simulink model "Tavola3_3ordine"  (R2018b)
settings: Solver=FixedStepAuto  StartTime=0.0  StopTime=70  RelTol=1e-3
libraries: simulink x1
settings Model: Creator=Utente  LastModifiedBy=giga4

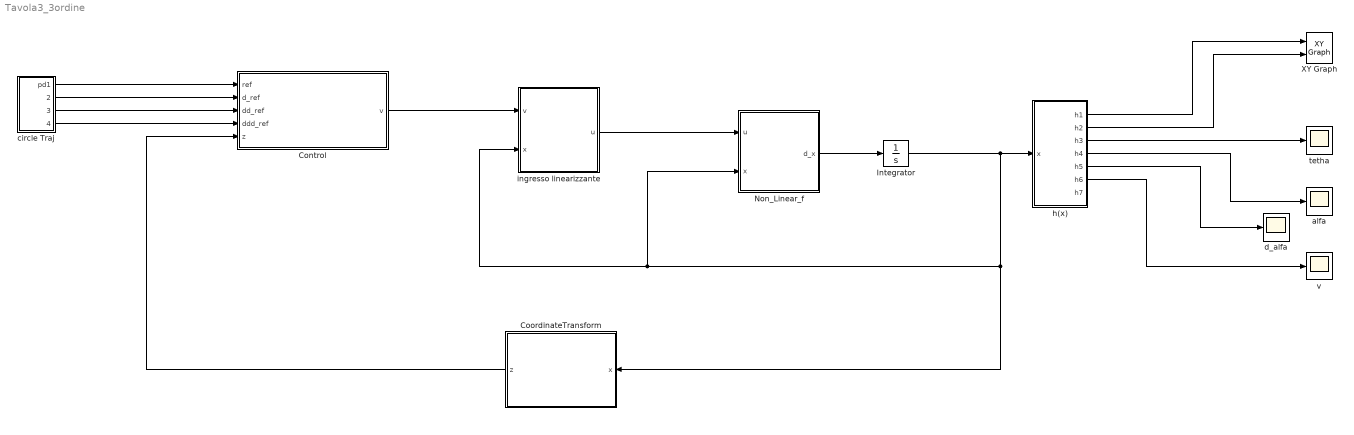
== system Tavola3_3ordine ==
  Control : MATLAB Function  TreatAsAtomicUnit=on
  CoordinateTransform : MATLAB Function  TreatAsAtomicUnit=on
  Integrator : Integrator  InitialCondition=[0,0,pi/2,0.017,0,5,0]
  "Non_Linear_f " : MATLAB Function  TreatAsAtomicUnit=on
  XY Graph : simulink/Sinks/XY Graph  xmin=-100  xmax=100  ymin=-100  ymax=100  st=-1
  alfa : Scope
  circle Traj : Subsystem
  d_alfa : Scope
  h(x) : MATLAB Function  TreatAsAtomicUnit=on
  ingresso linearizzante : MATLAB Function  TreatAsAtomicUnit=on
  tetha : Scope
  v : Scope
  wires:
  "Non_Linear_f "/1(d_x) -> Integrator/1
  Integrator/1 -> "Non_Linear_f "/2(x), ingresso linearizzante/2(x), CoordinateTransform/1(x), h(x)/1(x)
  ingresso linearizzante/1(u) -> "Non_Linear_f "/1(u)
  h(x)/3(h3) -> tetha/1
  h(x)/4(h4) -> alfa/1
  h(x)/1(h1) -> XY Graph/1
  h(x)/2(h2) -> XY Graph/2
  h(x)/6(h6) -> v/1
  Control/1(v) -> ingresso linearizzante/1(v)
  CoordinateTransform/1(z) -> Control/5(z)
  h(x)/5(h5) -> d_alfa/1
  circle Traj/1(pd1) -> Control/1(ref)
  circle Traj/2(d_pd1) -> Control/2(d_ref)
  circle Traj/3(dd_pd) -> Control/3(dd_ref)
  circle Traj/4(ddd_pd) -> Control/4(ddd_ref)

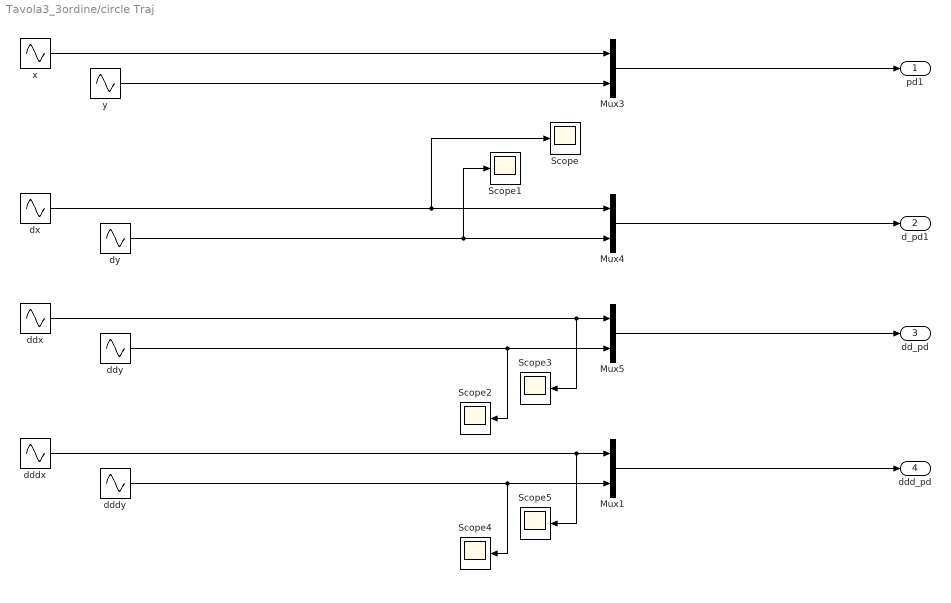
== system Tavola3_3ordine/circle Traj ==
  Mux{1,3..5} (4 alike) : Mux  Inputs=2
  Scope{,1..5} (6 alike) : Scope
  dddx : Sin  Amplitude=10  SampleTime=0
  dddy : Sin  Amplitude=-10  Phase=pi/2  SampleTime=0
  ddx : Sin  Amplitude=-10  Phase=pi/2  SampleTime=0
  ddy : Sin  Amplitude=-10  SampleTime=0
  dx : Sin  Amplitude=-10  SampleTime=0
  dy : Sin  Amplitude=10  Phase=pi/2  SampleTime=0
  x : Sin  Amplitude=10  Phase=pi/2  SampleTime=0
  y : Sin  Amplitude=10  SampleTime=0
  pd1 : Outport
  d_pd1 : Outport  Port=2
  dd_pd : Outport  Port=3
  ddd_pd : Outport  Port=4
  wires:
  ddx/1 -> Scope3/1, Mux5/1
  Mux3/1 -> pd1/1
  x/1 -> Mux3/1
  dddy/1 -> Scope4/1, Mux1/2
  ddy/1 -> Scope2/1, Mux5/2
  Mux1/1 -> ddd_pd/1
  dx/1 -> Scope/1, Mux4/1
  dy/1 -> Scope1/1, Mux4/2
  Mux5/1 -> dd_pd/1
  y/1 -> Mux3/2
  dddx/1 -> Scope5/1, Mux1/1
  Mux4/1 -> d_pd1/1

== matlab function Tavola3_3ordine/h(x) ==
  data: x input; h1 output; h2 output; h3 output; h4 output; h5 output; h6 output; h7 output
function [h1,h2,h3,h4,h5,h6,h7] = h(x)

x1 = x(1);
x2 = x(2);
x3 = x(3);
x4 = x(4);
x5 = x(5);
x6 = x(6);
x7 = x(7);


h1 = x1;
h2 = x2;
h3 = x3;
h4 = x4;
h5 = x5;
h6 = x6;
h7 = x7;

== matlab function Tavola3_3ordine/Non_Linear_f  ==
  data: u input; d_x output; x input
function d_x = statespacef(u,x)

x1 = x(1);
x2 = x(2);
x3 = x(3);
x4 = x(4);
x5 = x(5);
x6 = x(6);
x7 = x(7);


f =                                                                                                                               [x6*cos(x3);
                                                                                                                                  x6*sin(x3);
                                                                                                                                          x7;
                                                                                                                                          x5;
 (2.39*sin(2.0*x4)*x5^2)/(4.79*cos(x4)^2 - 12.5) - (173.0*sin(x4))/(4.79*cos(x4)^2 - 12.5) - (3.28*x7^2*sin(2.0*x4))/(4.79*cos(x4)^2 - 12.5);
       (1.99*sin(3.0*x4) - 6.77*sin(x4))*x7^2 + (23.5*sin(2.0*x4))/(4.79*cos(x4)^2 - 12.5) - (2.19*x5^2*sin(2.0*x4))/(4.79*cos(x4)^2 - 12.5);
                                       (0.547*x6*x7*sin(x4))/(0.228*cos(x4)^2 - 0.315) + (0.228*x5*x7*sin(2.0*x4))/(0.228*cos(x4)^2 - 0.315)];
g1 = [                                              0;
                                                    0;
                                                    0;
                                                    0;
        (2.19*cos(x3) + 3.11)/(4.79*cos(x4)^2 - 12.5);
 -(1.0*(0.547*cos(x4) + 1.0))/(4.79*cos(x4)^2 - 12.5);
                      -0.05/(0.228*cos(x4)^2 - 0.315);];
 
g2 = [                                              0;
                                                    0;
                                                    0;
                                                    0;
        (2.19*cos(x3) + 3.11)/(4.79*cos(x4)^2 - 12.5);
 -(1.0*(0.547*cos(x4) + 1.0))/(4.79*cos(x4)^2 - 12.5);
                       0.05/(0.228*cos(x4)^2 - 0.315)];
d_x = f + [g1,g2]*u;

== matlab function Tavola3_3ordine/ingresso linearizzante ==
  data: v input; u output; x input
function u = inputLinearizzante(v,x)

x1 = x(1);
x2 = x(2);
x3 = x(3);
x4 = x(4);
x5 = x(5);
x6 = x(6);
x7 = x(7);

inv_E =  [                                                                                                                                                                                     -(1.0*cos(x3)*(0.547*cos(x4) + 1.0))/(4.79*cos(x4)^2 - 12.5),                                                                                                                                                                                     -(1.0*cos(x3)*(0.547*cos(x4) + 1.0))/(4.79*cos(x4)^2 - 12.5);
          - (0.05*(x6*cos(x3) + 2*x7*sin(x3)*(1.99*sin(3.0*x4) - 6.77*sin(x4))))/(0.228*cos(x4)^2 - 0.315) - (1.0*x7*cos(x3)*(0.547*cos(x4) + 1.0))/(4.79*cos(x4)^2 - 12.5) - (4.38*x5*sin(2.0*x4)*sin(x3)*(2.19*cos(x3) + 3.11))/(4.79*cos(x4)^2 - 12.5)^2, (0.05*(x6*cos(x3) + 2*x7*sin(x3)*(1.99*sin(3.0*x4) - 6.77*sin(x4))))/(0.228*cos(x4)^2 - 0.315) - (1.0*x7*cos(x3)*(0.547*cos(x4) + 1.0))/(4.79*cos(x4)^2 - 12.5) - (4.38*x5*sin(2.0*x4)*sin(x3)*(2.19*cos(x3) + 3.11))/(4.79*cos(x4)^2 - 12.5)^2];
       
Gamma =  [                                                                                                                                                                                                                                                                                                                                                                                                                                                                                                                                                                                                                                                                                                                                                                                                                         cos(x3)*((1.99*sin(3.0*x4) - 6.77*sin(x4))*x7^2 + (23.5*sin(2.0*x4))/(4.79*cos(x4)^2 - 12.5) - (2.19*x5^2*sin(2.0*x4))/(4.79*cos(x4)^2 - 12.5)) - x6*x7*sin(x3);
 ((0.547*x6*x7*sin(x4))/(0.228*cos(x4)^2 - 0.315) + (0.228*x5*x7*sin(2.0*x4))/(0.228*cos(x4)^2 - 0.315))*(x6*cos(x3) + 2*x7*sin(x3)*(1.99*sin(3.0*x4) - 6.77*sin(x4))) + x7*(cos(x3)*((1.99*sin(3.0*x4) - 6.77*sin(x4))*x7^2 + (23.5*sin(2.0*x4))/(4.79*cos(x4)^2 - 12.5) - (2.19*x5^2*sin(2.0*x4))/(4.79*cos(x4)^2 - 12.5)) - x6*x7*sin(x3)) + x5*sin(x3)*(x7^2*(5.98*cos(3.0*x4) - 6.77*cos(x4)) + (46.9*cos(2.0*x4))/(4.79*cos(x4)^2 - 12.5) - (4.38*x5^2*cos(2.0*x4))/(4.79*cos(x4)^2 - 12.5) + (225.0*sin(2.0*x4)*cos(x4)*sin(x4))/(4.79*cos(x4)^2 - 12.5)^2 - (21.0*x5^2*sin(2.0*x4)*cos(x4)*sin(x4))/(4.79*cos(x4)^2 - 12.5)^2) + x7*cos(x3)*((1.99*sin(3.0*x4) - 6.77*sin(x4))*x7^2 + (23.5*sin(2.0*x4))/(4.79*cos(x4)^2 - 12.5) - (2.19*x5^2*sin(2.0*x4))/(4.79*cos(x4)^2 - 12.5)) + (4.38*x5*sin(2.0*x4)*sin(x3)*((3.28*sin(2.0*x4)*x7^2)/(4.79*cos(x4)^2 - 12.5) + (173.0*sin(x4))/(4.79*cos(x4)^2 - 12.5) - (2.39*x5^2*sin(2.0*x4))/(4.79*cos(x4)^2 - 12.5)))/(4.79*cos(x4)^2 - 12.5)];

 
 u = -inv_E*Gamma+inv_E*v;

== matlab function Tavola3_3ordine/CoordinateTransform ==
  data: z output; x input
function z = transformCoordinate(x)

x1 = x(1);
x2 = x(2);
x3 = x(3);
x4 = x(4);
x5 = x(5);
x6 = x(6);
x7 = x(7);

z =   [                                                                                                                                                       x1;
                                                                                                                                                      x6*cos(x3);
                                                                                                                                                              x2;
                                                                                                                                                      x6*sin(x3);
 sin(x3)*((1.99*sin(3.0*x4) - 6.77*sin(x4))*x7^2 + (23.5*sin(2.0*x4))/(4.79*cos(x4)^2 - 12.5) - (2.19*x5^2*sin(2.0*x4))/(4.79*cos(x4)^2 - 12.5)) + x6*x7*cos(x3);
                                                                                                                                                              x4;
                                                                                                                                                              x5;];

== matlab function Tavola3_3ordine/Control ==
  data: ref input; d_ref input; dd_ref input; ddd_ref input; v output; z input
function v = control(ref,d_ref,dd_ref,ddd_ref,z)

    z1 = z(1);
    z2 = z(2);
    z3 = z(3);
    z4 = z(4);
    z5 = z(5);
    z6 = z(6);
    z7 = z(7);

    ex = z1 - ref(1);
    d_ex = z2 - d_ref(1);
    d2_ex = dd_ref(1);
    d3_ex = 0;

    ey = z3 - ref(2);
    d_ey = z4 - d_ref(2);
    d2_ey = z5 - dd_ref(2);
    d3_ey = ddd_ref(2);
    
    k11 = 100;
    k12 = 10;
    
    k21 = 100;
    k22 = 10;
    k23 = 1;
    
%     v1 = d2_ex - (k11*ex + k12*d_ex);
%     v2 = d3_ey - (k21*ey + k22*d_ey + k23*d2_ey);
    v1 =
    v2 =
    
%     v1 = -k11*z6;
%     v2 = -k11*z;
%     
    v = [v1;v2];

end
